simulink model "Ladder_Model"  (R2021b)
settings: Solver=VariableStepAuto  StartTime=0.0  StopTime=0.00005  RelTol=1e-3
model workspace (MAT data in the model file):
  f = [1 10010011.009 20020021.018 30030031.027 40040041.036 50050051.045 60060061.0541 70070071.0631 80080081.0721 90090091.0811 100100101.09 110110111.099 ... (1000 elements, 1x1000)]
  f1 = 120
  fff : Simulink.Parameter (value not decoded)
undefined symbols (not defined in the file or in its folder): c0, ct0, ct1, ct2, ct3, ct4, cu, cv, frequence
libraries: spsSeriesRLCBranchLib x190, spsGroundLib x49, spsControlledVoltageSourceLib x6, spsImpedanceMeasurementLib x6, spspowerguiLib x1
(part 2 of 2)

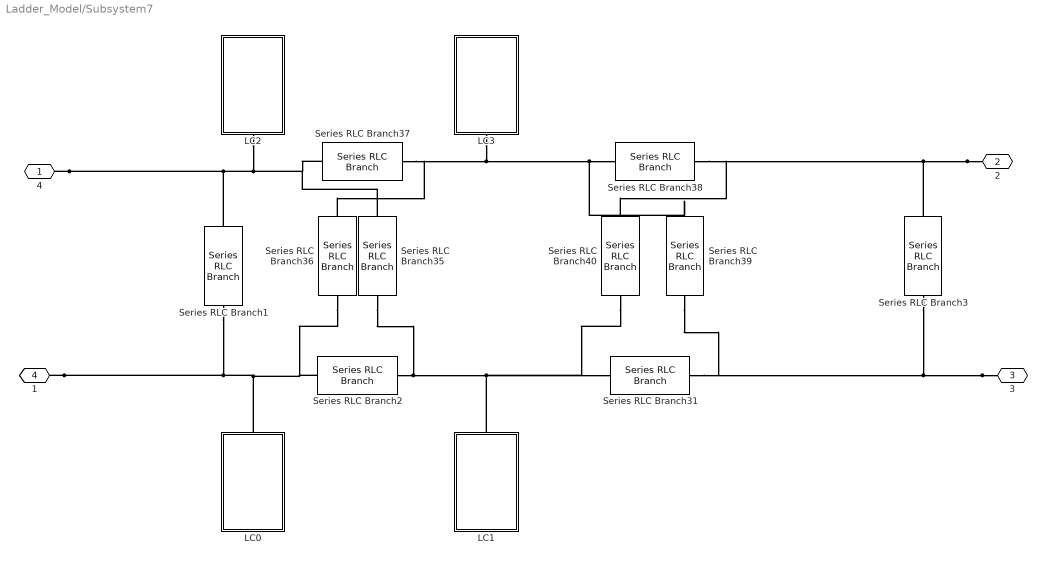
== system Ladder_Model/Subsystem7 ==
  LC0 : Subsystem
  LC1 : Subsystem
  LC2 : Subsystem
  LC3 : Subsystem
  Series RLC Branch1 : spsSeriesRLCBranchLib/Series RLC Branch  LConnTagsString=__new0  RConnTagsString=__new0  BranchType=C  Resistance=1  Inductance=1e-6  SetiL0=off  InitialCurrent=0  Capacitance=ct0  Setx0=off  InitialVoltage=0  Measurements=None
  Series RLC Branch2 : spsSeriesRLCBranchLib/Series RLC Branch  LConnTagsString=__new0  RConnTagsString=__new0  BranchType=C  Resistance=1  Inductance=1e-6  SetiL0=off  InitialCurrent=0  Capacitance=cu  Setx0=off  InitialVoltage=0  Measurements=None
  Series RLC Branch3 : spsSeriesRLCBranchLib/Series RLC Branch  LConnTagsString=__new0  RConnTagsString=__new0  BranchType=C  Resistance=1  Inductance=1e-6  SetiL0=off  InitialCurrent=0  Capacitance=ct0  Setx0=off  InitialVoltage=0  Measurements=None
  Series RLC Branch31 : spsSeriesRLCBranchLib/Series RLC Branch  LConnTagsString=__new0  RConnTagsString=__new0  BranchType=C  Resistance=1  Inductance=1e-6  SetiL0=off  InitialCurrent=0  Capacitance=cv  Setx0=off  InitialVoltage=0  Measurements=None
  Series RLC Branch35 : spsSeriesRLCBranchLib/Series RLC Branch  LConnTagsString=__new0  RConnTagsString=__new0  BranchType=C  Resistance=1  Inductance=1e-6  SetiL0=off  InitialCurrent=0  Capacitance=ct2  Setx0=off  InitialVoltage=0  Measurements=None
  Series RLC Branch36 : spsSeriesRLCBranchLib/Series RLC Branch  LConnTagsString=__new0  RConnTagsString=__new0  BranchType=C  Resistance=1  Inductance=1e-6  SetiL0=off  InitialCurrent=0  Capacitance=ct1  Setx0=off  InitialVoltage=0  Measurements=None
  Series RLC Branch37 : spsSeriesRLCBranchLib/Series RLC Branch  LConnTagsString=__new0  RConnTagsString=__new0  BranchType=C  Resistance=1  Inductance=1e-6  SetiL0=off  InitialCurrent=0  Capacitance=cu  Setx0=off  InitialVoltage=0  Measurements=None
  Series RLC Branch38 : spsSeriesRLCBranchLib/Series RLC Branch  LConnTagsString=__new0  RConnTagsString=__new0  BranchType=C  Resistance=1  Inductance=1e-6  SetiL0=off  InitialCurrent=0  Capacitance=cv  Setx0=off  InitialVoltage=0  Measurements=None
  Series RLC Branch39 : spsSeriesRLCBranchLib/Series RLC Branch  LConnTagsString=__new0  RConnTagsString=__new0  BranchType=C  Resistance=1  Inductance=1e-6  SetiL0=off  InitialCurrent=0  Capacitance=ct4  Setx0=off  InitialVoltage=0  Measurements=None
  Series RLC Branch40 : spsSeriesRLCBranchLib/Series RLC Branch  LConnTagsString=__new0  RConnTagsString=__new0  BranchType=C  Resistance=1  Inductance=1e-6  SetiL0=off  InitialCurrent=0  Capacitance=ct3  Setx0=off  InitialVoltage=0  Measurements=None
  4 : PMIOPort  Side=Left
  2 : PMIOPort  Port=2  Side=Right
  3 : PMIOPort  Port=3  Side=Right
  1 : PMIOPort  Port=4  Side=Left
  connections:
  3/RConn1 -- Series RLC Branch39/RConn1 -- Series RLC Branch31/RConn1 -- Series RLC Branch3/LConn1
  Series RLC Branch39/LConn1 -- Series RLC Branch38/LConn1 -- Series RLC Branch37/RConn1 -- Series RLC Branch36/RConn1 -- LC3/LConn1
  4/RConn1 -- Series RLC Branch37/LConn1 -- Series RLC Branch35/LConn1 -- LC2/LConn1 -- Series RLC Branch1/RConn1
  Series RLC Branch35/RConn1 -- Series RLC Branch2/RConn1 -- LC1/LConn1 -- Series RLC Branch40/LConn1 -- Series RLC Branch31/LConn1
  2/RConn1 -- Series RLC Branch40/RConn1 -- Series RLC Branch38/RConn1 -- Series RLC Branch3/RConn1
  1/RConn1 -- Series RLC Branch36/LConn1 -- Series RLC Branch2/LConn1 -- LC0/LConn1 -- Series RLC Branch1/LConn1

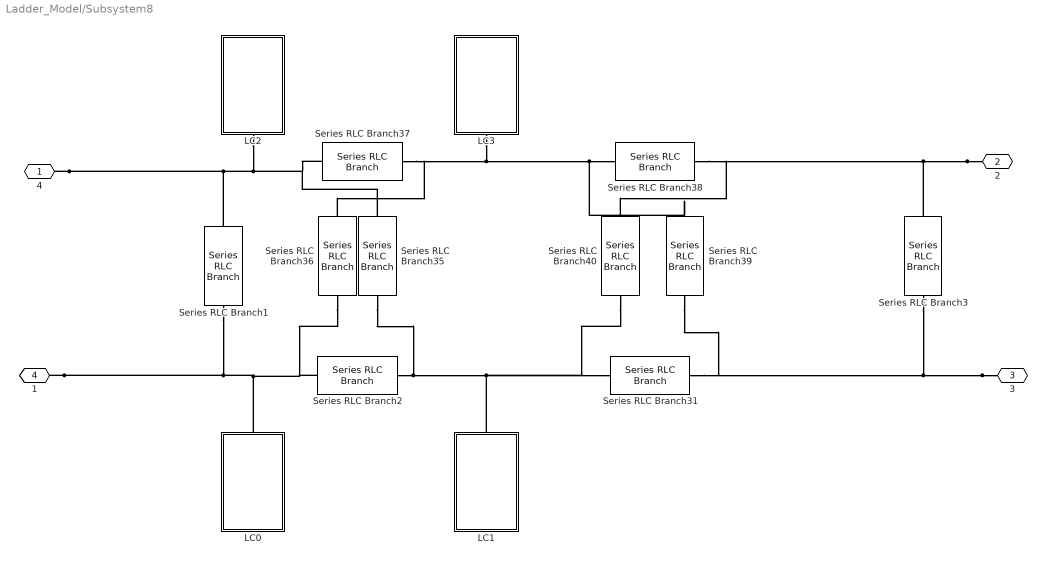
== system Ladder_Model/Subsystem8 ==
  LC0 : Subsystem
  LC1 : Subsystem
  LC2 : Subsystem
  LC3 : Subsystem
  Series RLC Branch1 : spsSeriesRLCBranchLib/Series RLC Branch  LConnTagsString=__new0  RConnTagsString=__new0  BranchType=C  Resistance=1  Inductance=1e-6  SetiL0=off  InitialCurrent=0  Capacitance=ct0  Setx0=off  InitialVoltage=0  Measurements=None
  Series RLC Branch2 : spsSeriesRLCBranchLib/Series RLC Branch  LConnTagsString=__new0  RConnTagsString=__new0  BranchType=C  Resistance=1  Inductance=1e-6  SetiL0=off  InitialCurrent=0  Capacitance=cu  Setx0=off  InitialVoltage=0  Measurements=None
  Series RLC Branch3 : spsSeriesRLCBranchLib/Series RLC Branch  LConnTagsString=__new0  RConnTagsString=__new0  BranchType=C  Resistance=1  Inductance=1e-6  SetiL0=off  InitialCurrent=0  Capacitance=ct0  Setx0=off  InitialVoltage=0  Measurements=None
  Series RLC Branch31 : spsSeriesRLCBranchLib/Series RLC Branch  LConnTagsString=__new0  RConnTagsString=__new0  BranchType=C  Resistance=1  Inductance=1e-6  SetiL0=off  InitialCurrent=0  Capacitance=cv  Setx0=off  InitialVoltage=0  Measurements=None
  Series RLC Branch35 : spsSeriesRLCBranchLib/Series RLC Branch  LConnTagsString=__new0  RConnTagsString=__new0  BranchType=C  Resistance=1  Inductance=1e-6  SetiL0=off  InitialCurrent=0  Capacitance=ct2  Setx0=off  InitialVoltage=0  Measurements=None
  Series RLC Branch36 : spsSeriesRLCBranchLib/Series RLC Branch  LConnTagsString=__new0  RConnTagsString=__new0  BranchType=C  Resistance=1  Inductance=1e-6  SetiL0=off  InitialCurrent=0  Capacitance=ct1  Setx0=off  InitialVoltage=0  Measurements=None
  Series RLC Branch37 : spsSeriesRLCBranchLib/Series RLC Branch  LConnTagsString=__new0  RConnTagsString=__new0  BranchType=C  Resistance=1  Inductance=1e-6  SetiL0=off  InitialCurrent=0  Capacitance=cu  Setx0=off  InitialVoltage=0  Measurements=None
  Series RLC Branch38 : spsSeriesRLCBranchLib/Series RLC Branch  LConnTagsString=__new0  RConnTagsString=__new0  BranchType=C  Resistance=1  Inductance=1e-6  SetiL0=off  InitialCurrent=0  Capacitance=cv  Setx0=off  InitialVoltage=0  Measurements=None
  Series RLC Branch39 : spsSeriesRLCBranchLib/Series RLC Branch  LConnTagsString=__new0  RConnTagsString=__new0  BranchType=C  Resistance=1  Inductance=1e-6  SetiL0=off  InitialCurrent=0  Capacitance=ct4  Setx0=off  InitialVoltage=0  Measurements=None
  Series RLC Branch40 : spsSeriesRLCBranchLib/Series RLC Branch  LConnTagsString=__new0  RConnTagsString=__new0  BranchType=C  Resistance=1  Inductance=1e-6  SetiL0=off  InitialCurrent=0  Capacitance=ct3  Setx0=off  InitialVoltage=0  Measurements=None
  4 : PMIOPort  Side=Left
  2 : PMIOPort  Port=2  Side=Right
  3 : PMIOPort  Port=3  Side=Right
  1 : PMIOPort  Port=4  Side=Left
  connections:
  3/RConn1 -- Series RLC Branch39/RConn1 -- Series RLC Branch31/RConn1 -- Series RLC Branch3/LConn1
  Series RLC Branch39/LConn1 -- Series RLC Branch38/LConn1 -- Series RLC Branch37/RConn1 -- Series RLC Branch36/RConn1 -- LC3/LConn1
  4/RConn1 -- Series RLC Branch37/LConn1 -- Series RLC Branch35/LConn1 -- LC2/LConn1 -- Series RLC Branch1/RConn1
  Series RLC Branch35/RConn1 -- Series RLC Branch2/RConn1 -- LC1/LConn1 -- Series RLC Branch40/LConn1 -- Series RLC Branch31/LConn1
  2/RConn1 -- Series RLC Branch40/RConn1 -- Series RLC Branch38/RConn1 -- Series RLC Branch3/RConn1
  1/RConn1 -- Series RLC Branch36/LConn1 -- Series RLC Branch2/LConn1 -- LC0/LConn1 -- Series RLC Branch1/LConn1

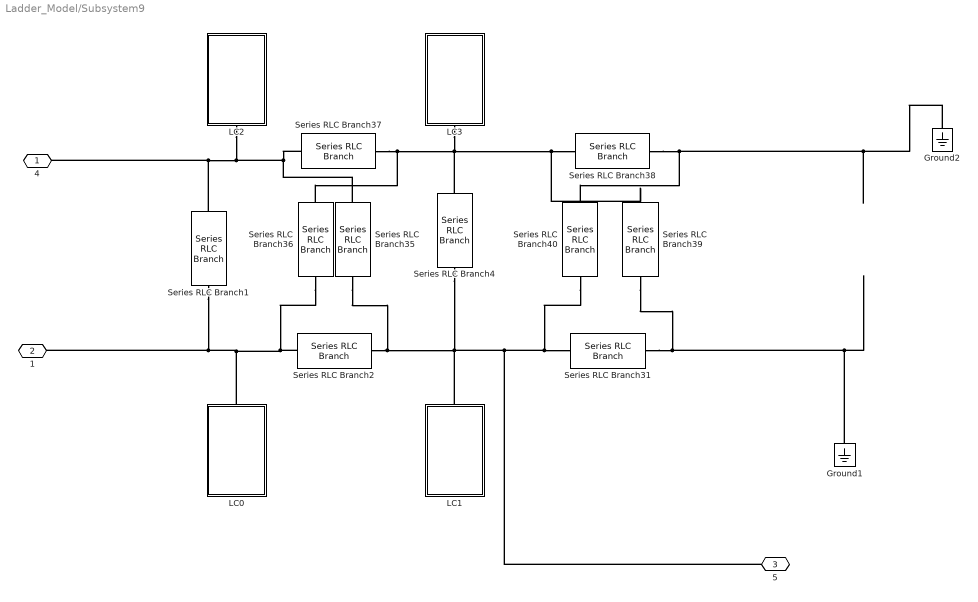
== system Ladder_Model/Subsystem9 ==
  Ground1 : spsGroundLib/Ground  LConnTagsString=a
  Ground2 : spsGroundLib/Ground  LConnTagsString=a
  LC0 : Subsystem
  LC1 : Subsystem
  LC2 : Subsystem
  LC3 : Subsystem
  Series RLC Branch1 : spsSeriesRLCBranchLib/Series RLC Branch  LConnTagsString=__new0  RConnTagsString=__new0  BranchType=C  Resistance=1  Inductance=1e-6  SetiL0=off  InitialCurrent=0  Capacitance=ct0  Setx0=off  InitialVoltage=0  Measurements=None
  Series RLC Branch2 : spsSeriesRLCBranchLib/Series RLC Branch  LConnTagsString=__new0  RConnTagsString=__new0  BranchType=C  Resistance=1  Inductance=1e-6  SetiL0=off  InitialCurrent=0  Capacitance=cu  Setx0=off  InitialVoltage=0  Measurements=None
  Series RLC Branch31 : spsSeriesRLCBranchLib/Series RLC Branch  LConnTagsString=__new0  RConnTagsString=__new0  BranchType=C  Resistance=1  Inductance=1e-6  SetiL0=off  InitialCurrent=0  Capacitance=cv  Setx0=off  InitialVoltage=0  Measurements=None
  Series RLC Branch35 : spsSeriesRLCBranchLib/Series RLC Branch  LConnTagsString=__new0  RConnTagsString=__new0  BranchType=C  Resistance=1  Inductance=1e-6  SetiL0=off  InitialCurrent=0  Capacitance=ct2  Setx0=off  InitialVoltage=0  Measurements=None
  Series RLC Branch36 : spsSeriesRLCBranchLib/Series RLC Branch  LConnTagsString=__new0  RConnTagsString=__new0  BranchType=C  Resistance=1  Inductance=1e-6  SetiL0=off  InitialCurrent=0  Capacitance=ct1  Setx0=off  InitialVoltage=0  Measurements=None
  Series RLC Branch37 : spsSeriesRLCBranchLib/Series RLC Branch  LConnTagsString=__new0  RConnTagsString=__new0  BranchType=C  Resistance=1  Inductance=1e-6  SetiL0=off  InitialCurrent=0  Capacitance=cu  Setx0=off  InitialVoltage=0  Measurements=None
  Series RLC Branch38 : spsSeriesRLCBranchLib/Series RLC Branch  LConnTagsString=__new0  RConnTagsString=__new0  BranchType=C  Resistance=1  Inductance=1e-6  SetiL0=off  InitialCurrent=0  Capacitance=cv  Setx0=off  InitialVoltage=0  Measurements=None
  Series RLC Branch39 : spsSeriesRLCBranchLib/Series RLC Branch  LConnTagsString=__new0  RConnTagsString=__new0  BranchType=C  Resistance=1  Inductance=1e-6  SetiL0=off  InitialCurrent=0  Capacitance=ct4  Setx0=off  InitialVoltage=0  Measurements=None
  Series RLC Branch4 : spsSeriesRLCBranchLib/Series RLC Branch  LConnTagsString=__new0  RConnTagsString=__new0  BranchType=C  Resistance=1  Inductance=1e-6  SetiL0=off  InitialCurrent=0  Capacitance=ct0  Setx0=off  InitialVoltage=0  Measurements=None
  Series RLC Branch40 : spsSeriesRLCBranchLib/Series RLC Branch  LConnTagsString=__new0  RConnTagsString=__new0  BranchType=C  Resistance=1  Inductance=1e-6  SetiL0=off  InitialCurrent=0  Capacitance=ct3  Setx0=off  InitialVoltage=0  Measurements=None
  4 : PMIOPort  Side=Left
  1 : PMIOPort  Port=2  Side=Left
  5 : PMIOPort  Port=3  Side=Right
  connections:
  Series RLC Branch39/RConn1 -- Ground1/LConn1 -- Series RLC Branch31/RConn1
  Series RLC Branch39/LConn1 -- Series RLC Branch4/RConn1 -- Series RLC Branch37/RConn1 -- Series RLC Branch36/RConn1 -- LC3/LConn1 -- Series RLC Branch38/LConn1
  4/RConn1 -- Series RLC Branch37/LConn1 -- Series RLC Branch35/LConn1 -- LC2/LConn1 -- Series RLC Branch1/RConn1
  Series RLC Branch35/RConn1 -- Series RLC Branch2/RConn1 -- Series RLC Branch4/LConn1 -- 5/RConn1 -- Series RLC Branch40/LConn1 -- Series RLC Branch31/LConn1 -- LC1/LConn1
  Series RLC Branch40/RConn1 -- Ground2/LConn1 -- Series RLC Branch38/RConn1
  1/RConn1 -- Series RLC Branch36/LConn1 -- Series RLC Branch2/LConn1 -- LC0/LConn1 -- Series RLC Branch1/LConn1

== system Ladder_Model/Subsystem/LC0 ==
  Ground : spsGroundLib/Ground  LConnTagsString=a
  Series RLC Branch2 : spsSeriesRLCBranchLib/Series RLC Branch  LConnTagsString=__new0  RConnTagsString=__new0  BranchType=L  Resistance=1  Inductance=1e-6  SetiL0=off  InitialCurrent=0  Capacitance=1e-6  Setx0=off  InitialVoltage=0  Measurements=None
  Series RLC Branch31 : spsSeriesRLCBranchLib/Series RLC Branch  LConnTagsString=__new0  RConnTagsString=__new0  BranchType=C  Resistance=1  Inductance=1e-6  SetiL0=off  InitialCurrent=0  Capacitance=c0  Setx0=off  InitialVoltage=0  Measurements=None
  Conn1 : PMIOPort  Side=Left
  connections:
  Series RLC Branch2/LConn1 -- Conn1/RConn1 -- Series RLC Branch31/LConn1
  Series RLC Branch2/RConn1 -- Ground/LConn1 -- Series RLC Branch31/RConn1

== system Ladder_Model/Subsystem/LC1 ==
  Ground : spsGroundLib/Ground  LConnTagsString=a
  Series RLC Branch2 : spsSeriesRLCBranchLib/Series RLC Branch  LConnTagsString=__new0  RConnTagsString=__new0  BranchType=L  Resistance=1  Inductance=1e-6  SetiL0=off  InitialCurrent=0  Capacitance=1e-6  Setx0=off  InitialVoltage=0  Measurements=None
  Series RLC Branch31 : spsSeriesRLCBranchLib/Series RLC Branch  LConnTagsString=__new0  RConnTagsString=__new0  BranchType=C  Resistance=1  Inductance=1e-6  SetiL0=off  InitialCurrent=0  Capacitance=c0  Setx0=off  InitialVoltage=0  Measurements=None
  Conn1 : PMIOPort  Side=Left
  connections:
  Series RLC Branch31/LConn1 -- Series RLC Branch2/LConn1 -- Conn1/RConn1
  Series RLC Branch31/RConn1 -- Series RLC Branch2/RConn1 -- Ground/LConn1

== system Ladder_Model/Subsystem/LC2 ==
  Ground : spsGroundLib/Ground  LConnTagsString=a
  Series RLC Branch2 : spsSeriesRLCBranchLib/Series RLC Branch  LConnTagsString=__new0  RConnTagsString=__new0  BranchType=L  Resistance=1  Inductance=1e-6  SetiL0=off  InitialCurrent=0  Capacitance=1e-6  Setx0=off  InitialVoltage=0  Measurements=None
  Series RLC Branch31 : spsSeriesRLCBranchLib/Series RLC Branch  LConnTagsString=__new0  RConnTagsString=__new0  BranchType=C  Resistance=1  Inductance=1e-6  SetiL0=off  InitialCurrent=0  Capacitance=c0  Setx0=off  InitialVoltage=0  Measurements=None
  Conn1 : PMIOPort  Side=Left
  connections:
  Series RLC Branch31/LConn1 -- Series RLC Branch2/LConn1 -- Conn1/RConn1
  Series RLC Branch31/RConn1 -- Series RLC Branch2/RConn1 -- Ground/LConn1

== system Ladder_Model/Subsystem/LC3 ==
  Ground : spsGroundLib/Ground  LConnTagsString=a
  Series RLC Branch2 : spsSeriesRLCBranchLib/Series RLC Branch  LConnTagsString=__new0  RConnTagsString=__new0  BranchType=L  Resistance=1  Inductance=1e-6  SetiL0=off  InitialCurrent=0  Capacitance=1e-6  Setx0=off  InitialVoltage=0  Measurements=None
  Series RLC Branch31 : spsSeriesRLCBranchLib/Series RLC Branch  LConnTagsString=__new0  RConnTagsString=__new0  BranchType=C  Resistance=1  Inductance=1e-6  SetiL0=off  InitialCurrent=0  Capacitance=c0  Setx0=off  InitialVoltage=0  Measurements=None
  Conn1 : PMIOPort  Side=Left
  connections:
  Series RLC Branch31/LConn1 -- Series RLC Branch2/LConn1 -- Conn1/RConn1
  Series RLC Branch31/RConn1 -- Series RLC Branch2/RConn1 -- Ground/LConn1

== system Ladder_Model/Subsystem1/LC0 ==
  Ground : spsGroundLib/Ground  LConnTagsString=a
  Series RLC Branch2 : spsSeriesRLCBranchLib/Series RLC Branch  LConnTagsString=__new0  RConnTagsString=__new0  BranchType=L  Resistance=1  Inductance=1e-6  SetiL0=off  InitialCurrent=0  Capacitance=1e-6  Setx0=off  InitialVoltage=0  Measurements=None
  Series RLC Branch31 : spsSeriesRLCBranchLib/Series RLC Branch  LConnTagsString=__new0  RConnTagsString=__new0  BranchType=C  Resistance=1  Inductance=1e-6  SetiL0=off  InitialCurrent=0  Capacitance=c0  Setx0=off  InitialVoltage=0  Measurements=None
  Conn1 : PMIOPort  Side=Left
  connections:
  Series RLC Branch31/LConn1 -- Series RLC Branch2/LConn1 -- Conn1/RConn1
  Series RLC Branch31/RConn1 -- Series RLC Branch2/RConn1 -- Ground/LConn1

== system Ladder_Model/Subsystem1/LC1 ==
  Ground : spsGroundLib/Ground  LConnTagsString=a
  Series RLC Branch2 : spsSeriesRLCBranchLib/Series RLC Branch  LConnTagsString=__new0  RConnTagsString=__new0  BranchType=L  Resistance=1  Inductance=1e-6  SetiL0=off  InitialCurrent=0  Capacitance=1e-6  Setx0=off  InitialVoltage=0  Measurements=None
  Series RLC Branch31 : spsSeriesRLCBranchLib/Series RLC Branch  LConnTagsString=__new0  RConnTagsString=__new0  BranchType=C  Resistance=1  Inductance=1e-6  SetiL0=off  InitialCurrent=0  Capacitance=c0  Setx0=off  InitialVoltage=0  Measurements=None
  Conn1 : PMIOPort  Side=Left
  connections:
  Series RLC Branch31/LConn1 -- Series RLC Branch2/LConn1 -- Conn1/RConn1
  Series RLC Branch31/RConn1 -- Series RLC Branch2/RConn1 -- Ground/LConn1

== system Ladder_Model/Subsystem1/LC2 ==
  Ground : spsGroundLib/Ground  LConnTagsString=a
  Series RLC Branch2 : spsSeriesRLCBranchLib/Series RLC Branch  LConnTagsString=__new0  RConnTagsString=__new0  BranchType=L  Resistance=1  Inductance=1e-6  SetiL0=off  InitialCurrent=0  Capacitance=1e-6  Setx0=off  InitialVoltage=0  Measurements=None
  Series RLC Branch31 : spsSeriesRLCBranchLib/Series RLC Branch  LConnTagsString=__new0  RConnTagsString=__new0  BranchType=C  Resistance=1  Inductance=1e-6  SetiL0=off  InitialCurrent=0  Capacitance=c0  Setx0=off  InitialVoltage=0  Measurements=None
  Conn1 : PMIOPort  Side=Left
  connections:
  Series RLC Branch31/LConn1 -- Series RLC Branch2/LConn1 -- Conn1/RConn1
  Series RLC Branch31/RConn1 -- Series RLC Branch2/RConn1 -- Ground/LConn1

== system Ladder_Model/Subsystem1/LC3 ==
  Ground : spsGroundLib/Ground  LConnTagsString=a
  Series RLC Branch2 : spsSeriesRLCBranchLib/Series RLC Branch  LConnTagsString=__new0  RConnTagsString=__new0  BranchType=L  Resistance=1  Inductance=1e-6  SetiL0=off  InitialCurrent=0  Capacitance=1e-6  Setx0=off  InitialVoltage=0  Measurements=None
  Series RLC Branch31 : spsSeriesRLCBranchLib/Series RLC Branch  LConnTagsString=__new0  RConnTagsString=__new0  BranchType=C  Resistance=1  Inductance=1e-6  SetiL0=off  InitialCurrent=0  Capacitance=c0  Setx0=off  InitialVoltage=0  Measurements=None
  Conn1 : PMIOPort  Side=Left
  connections:
  Series RLC Branch31/LConn1 -- Series RLC Branch2/LConn1 -- Conn1/RConn1
  Series RLC Branch31/RConn1 -- Series RLC Branch2/RConn1 -- Ground/LConn1

== system Ladder_Model/Subsystem2/LC0 ==
  Ground : spsGroundLib/Ground  LConnTagsString=a
  Series RLC Branch2 : spsSeriesRLCBranchLib/Series RLC Branch  LConnTagsString=__new0  RConnTagsString=__new0  BranchType=L  Resistance=1  Inductance=1e-6  SetiL0=off  InitialCurrent=0  Capacitance=1e-6  Setx0=off  InitialVoltage=0  Measurements=None
  Series RLC Branch31 : spsSeriesRLCBranchLib/Series RLC Branch  LConnTagsString=__new0  RConnTagsString=__new0  BranchType=C  Resistance=1  Inductance=1e-6  SetiL0=off  InitialCurrent=0  Capacitance=c0  Setx0=off  InitialVoltage=0  Measurements=None
  Conn1 : PMIOPort  Side=Left
  connections:
  Series RLC Branch31/LConn1 -- Series RLC Branch2/LConn1 -- Conn1/RConn1
  Series RLC Branch31/RConn1 -- Series RLC Branch2/RConn1 -- Ground/LConn1

== system Ladder_Model/Subsystem2/LC1 ==
  Ground : spsGroundLib/Ground  LConnTagsString=a
  Series RLC Branch2 : spsSeriesRLCBranchLib/Series RLC Branch  LConnTagsString=__new0  RConnTagsString=__new0  BranchType=L  Resistance=1  Inductance=1e-6  SetiL0=off  InitialCurrent=0  Capacitance=1e-6  Setx0=off  InitialVoltage=0  Measurements=None
  Series RLC Branch31 : spsSeriesRLCBranchLib/Series RLC Branch  LConnTagsString=__new0  RConnTagsString=__new0  BranchType=C  Resistance=1  Inductance=1e-6  SetiL0=off  InitialCurrent=0  Capacitance=c0  Setx0=off  InitialVoltage=0  Measurements=None
  Conn1 : PMIOPort  Side=Left
  connections:
  Series RLC Branch31/LConn1 -- Series RLC Branch2/LConn1 -- Conn1/RConn1
  Series RLC Branch31/RConn1 -- Series RLC Branch2/RConn1 -- Ground/LConn1

== system Ladder_Model/Subsystem2/LC2 ==
  Ground : spsGroundLib/Ground  LConnTagsString=a
  Series RLC Branch2 : spsSeriesRLCBranchLib/Series RLC Branch  LConnTagsString=__new0  RConnTagsString=__new0  BranchType=L  Resistance=1  Inductance=1e-6  SetiL0=off  InitialCurrent=0  Capacitance=1e-6  Setx0=off  InitialVoltage=0  Measurements=None
  Series RLC Branch31 : spsSeriesRLCBranchLib/Series RLC Branch  LConnTagsString=__new0  RConnTagsString=__new0  BranchType=C  Resistance=1  Inductance=1e-6  SetiL0=off  InitialCurrent=0  Capacitance=c0  Setx0=off  InitialVoltage=0  Measurements=None
  Conn1 : PMIOPort  Side=Left
  connections:
  Series RLC Branch31/LConn1 -- Series RLC Branch2/LConn1 -- Conn1/RConn1
  Series RLC Branch31/RConn1 -- Series RLC Branch2/RConn1 -- Ground/LConn1

== system Ladder_Model/Subsystem2/LC3 ==
  Ground : spsGroundLib/Ground  LConnTagsString=a
  Series RLC Branch2 : spsSeriesRLCBranchLib/Series RLC Branch  LConnTagsString=__new0  RConnTagsString=__new0  BranchType=L  Resistance=1  Inductance=1e-6  SetiL0=off  InitialCurrent=0  Capacitance=1e-6  Setx0=off  InitialVoltage=0  Measurements=None
  Series RLC Branch31 : spsSeriesRLCBranchLib/Series RLC Branch  LConnTagsString=__new0  RConnTagsString=__new0  BranchType=C  Resistance=1  Inductance=1e-6  SetiL0=off  InitialCurrent=0  Capacitance=c0  Setx0=off  InitialVoltage=0  Measurements=None
  Conn1 : PMIOPort  Side=Left
  connections:
  Series RLC Branch31/LConn1 -- Series RLC Branch2/LConn1 -- Conn1/RConn1
  Series RLC Branch31/RConn1 -- Series RLC Branch2/RConn1 -- Ground/LConn1

== system Ladder_Model/Subsystem3/LC0 ==
  Ground : spsGroundLib/Ground  LConnTagsString=a
  Series RLC Branch2 : spsSeriesRLCBranchLib/Series RLC Branch  LConnTagsString=__new0  RConnTagsString=__new0  BranchType=L  Resistance=1  Inductance=1e-6  SetiL0=off  InitialCurrent=0  Capacitance=1e-6  Setx0=off  InitialVoltage=0  Measurements=None
  Series RLC Branch31 : spsSeriesRLCBranchLib/Series RLC Branch  LConnTagsString=__new0  RConnTagsString=__new0  BranchType=C  Resistance=1  Inductance=1e-6  SetiL0=off  InitialCurrent=0  Capacitance=c0  Setx0=off  InitialVoltage=0  Measurements=None
  Conn1 : PMIOPort  Side=Left
  connections:
  Series RLC Branch31/LConn1 -- Series RLC Branch2/LConn1 -- Conn1/RConn1
  Series RLC Branch31/RConn1 -- Series RLC Branch2/RConn1 -- Ground/LConn1

== system Ladder_Model/Subsystem3/LC1 ==
  Ground : spsGroundLib/Ground  LConnTagsString=a
  Series RLC Branch2 : spsSeriesRLCBranchLib/Series RLC Branch  LConnTagsString=__new0  RConnTagsString=__new0  BranchType=L  Resistance=1  Inductance=1e-6  SetiL0=off  InitialCurrent=0  Capacitance=1e-6  Setx0=off  InitialVoltage=0  Measurements=None
  Series RLC Branch31 : spsSeriesRLCBranchLib/Series RLC Branch  LConnTagsString=__new0  RConnTagsString=__new0  BranchType=C  Resistance=1  Inductance=1e-6  SetiL0=off  InitialCurrent=0  Capacitance=c0  Setx0=off  InitialVoltage=0  Measurements=None
  Conn1 : PMIOPort  Side=Left
  connections:
  Series RLC Branch31/LConn1 -- Series RLC Branch2/LConn1 -- Conn1/RConn1
  Series RLC Branch31/RConn1 -- Series RLC Branch2/RConn1 -- Ground/LConn1

== system Ladder_Model/Subsystem3/LC2 ==
  Ground : spsGroundLib/Ground  LConnTagsString=a
  Series RLC Branch2 : spsSeriesRLCBranchLib/Series RLC Branch  LConnTagsString=__new0  RConnTagsString=__new0  BranchType=L  Resistance=1  Inductance=1e-6  SetiL0=off  InitialCurrent=0  Capacitance=1e-6  Setx0=off  InitialVoltage=0  Measurements=None
  Series RLC Branch31 : spsSeriesRLCBranchLib/Series RLC Branch  LConnTagsString=__new0  RConnTagsString=__new0  BranchType=C  Resistance=1  Inductance=1e-6  SetiL0=off  InitialCurrent=0  Capacitance=c0  Setx0=off  InitialVoltage=0  Measurements=None
  Conn1 : PMIOPort  Side=Left
  connections:
  Series RLC Branch31/LConn1 -- Series RLC Branch2/LConn1 -- Conn1/RConn1
  Series RLC Branch31/RConn1 -- Series RLC Branch2/RConn1 -- Ground/LConn1

== system Ladder_Model/Subsystem3/LC3 ==
  Ground : spsGroundLib/Ground  LConnTagsString=a
  Series RLC Branch2 : spsSeriesRLCBranchLib/Series RLC Branch  LConnTagsString=__new0  RConnTagsString=__new0  BranchType=L  Resistance=1  Inductance=1e-6  SetiL0=off  InitialCurrent=0  Capacitance=1e-6  Setx0=off  InitialVoltage=0  Measurements=None
  Series RLC Branch31 : spsSeriesRLCBranchLib/Series RLC Branch  LConnTagsString=__new0  RConnTagsString=__new0  BranchType=C  Resistance=1  Inductance=1e-6  SetiL0=off  InitialCurrent=0  Capacitance=c0  Setx0=off  InitialVoltage=0  Measurements=None
  Conn1 : PMIOPort  Side=Left
  connections:
  Series RLC Branch31/LConn1 -- Series RLC Branch2/LConn1 -- Conn1/RConn1
  Series RLC Branch31/RConn1 -- Series RLC Branch2/RConn1 -- Ground/LConn1

== system Ladder_Model/Subsystem4/LC0 ==
  Ground : spsGroundLib/Ground  LConnTagsString=a
  Series RLC Branch2 : spsSeriesRLCBranchLib/Series RLC Branch  LConnTagsString=__new0  RConnTagsString=__new0  BranchType=L  Resistance=1  Inductance=1e-6  SetiL0=off  InitialCurrent=0  Capacitance=1e-6  Setx0=off  InitialVoltage=0  Measurements=None
  Series RLC Branch31 : spsSeriesRLCBranchLib/Series RLC Branch  LConnTagsString=__new0  RConnTagsString=__new0  BranchType=C  Resistance=1  Inductance=1e-6  SetiL0=off  InitialCurrent=0  Capacitance=c0  Setx0=off  InitialVoltage=0  Measurements=None
  Conn1 : PMIOPort  Side=Left
  connections:
  Series RLC Branch31/LConn1 -- Series RLC Branch2/LConn1 -- Conn1/RConn1
  Series RLC Branch31/RConn1 -- Series RLC Branch2/RConn1 -- Ground/LConn1

== system Ladder_Model/Subsystem4/LC1 ==
  Ground : spsGroundLib/Ground  LConnTagsString=a
  Series RLC Branch2 : spsSeriesRLCBranchLib/Series RLC Branch  LConnTagsString=__new0  RConnTagsString=__new0  BranchType=L  Resistance=1  Inductance=1e-6  SetiL0=off  InitialCurrent=0  Capacitance=1e-6  Setx0=off  InitialVoltage=0  Measurements=None
  Series RLC Branch31 : spsSeriesRLCBranchLib/Series RLC Branch  LConnTagsString=__new0  RConnTagsString=__new0  BranchType=C  Resistance=1  Inductance=1e-6  SetiL0=off  InitialCurrent=0  Capacitance=c0  Setx0=off  InitialVoltage=0  Measurements=None
  Conn1 : PMIOPort  Side=Left
  connections:
  Series RLC Branch31/LConn1 -- Series RLC Branch2/LConn1 -- Conn1/RConn1
  Series RLC Branch31/RConn1 -- Series RLC Branch2/RConn1 -- Ground/LConn1

== system Ladder_Model/Subsystem4/LC2 ==
  Ground : spsGroundLib/Ground  LConnTagsString=a
  Series RLC Branch2 : spsSeriesRLCBranchLib/Series RLC Branch  LConnTagsString=__new0  RConnTagsString=__new0  BranchType=L  Resistance=1  Inductance=1e-6  SetiL0=off  InitialCurrent=0  Capacitance=1e-6  Setx0=off  InitialVoltage=0  Measurements=None
  Series RLC Branch31 : spsSeriesRLCBranchLib/Series RLC Branch  LConnTagsString=__new0  RConnTagsString=__new0  BranchType=C  Resistance=1  Inductance=1e-6  SetiL0=off  InitialCurrent=0  Capacitance=c0  Setx0=off  InitialVoltage=0  Measurements=None
  Conn1 : PMIOPort  Side=Left
  connections:
  Series RLC Branch31/LConn1 -- Series RLC Branch2/LConn1 -- Conn1/RConn1
  Series RLC Branch31/RConn1 -- Series RLC Branch2/RConn1 -- Ground/LConn1

== system Ladder_Model/Subsystem4/LC3 ==
  Ground : spsGroundLib/Ground  LConnTagsString=a
  Series RLC Branch2 : spsSeriesRLCBranchLib/Series RLC Branch  LConnTagsString=__new0  RConnTagsString=__new0  BranchType=L  Resistance=1  Inductance=1e-6  SetiL0=off  InitialCurrent=0  Capacitance=1e-6  Setx0=off  InitialVoltage=0  Measurements=None
  Series RLC Branch31 : spsSeriesRLCBranchLib/Series RLC Branch  LConnTagsString=__new0  RConnTagsString=__new0  BranchType=C  Resistance=1  Inductance=1e-6  SetiL0=off  InitialCurrent=0  Capacitance=c0  Setx0=off  InitialVoltage=0  Measurements=None
  Conn1 : PMIOPort  Side=Left
  connections:
  Series RLC Branch31/LConn1 -- Series RLC Branch2/LConn1 -- Conn1/RConn1
  Series RLC Branch31/RConn1 -- Series RLC Branch2/RConn1 -- Ground/LConn1

== system Ladder_Model/Subsystem5/LC0 ==
  Ground : spsGroundLib/Ground  LConnTagsString=a
  Series RLC Branch2 : spsSeriesRLCBranchLib/Series RLC Branch  LConnTagsString=__new0  RConnTagsString=__new0  BranchType=L  Resistance=1  Inductance=1e-6  SetiL0=off  InitialCurrent=0  Capacitance=1e-6  Setx0=off  InitialVoltage=0  Measurements=None
  Series RLC Branch31 : spsSeriesRLCBranchLib/Series RLC Branch  LConnTagsString=__new0  RConnTagsString=__new0  BranchType=C  Resistance=1  Inductance=1e-6  SetiL0=off  InitialCurrent=0  Capacitance=c0  Setx0=off  InitialVoltage=0  Measurements=None
  Conn1 : PMIOPort  Side=Left
  connections:
  Series RLC Branch31/LConn1 -- Series RLC Branch2/LConn1 -- Conn1/RConn1
  Series RLC Branch31/RConn1 -- Series RLC Branch2/RConn1 -- Ground/LConn1

== system Ladder_Model/Subsystem5/LC1 ==
  Ground : spsGroundLib/Ground  LConnTagsString=a
  Series RLC Branch2 : spsSeriesRLCBranchLib/Series RLC Branch  LConnTagsString=__new0  RConnTagsString=__new0  BranchType=L  Resistance=1  Inductance=1e-6  SetiL0=off  InitialCurrent=0  Capacitance=1e-6  Setx0=off  InitialVoltage=0  Measurements=None
  Series RLC Branch31 : spsSeriesRLCBranchLib/Series RLC Branch  LConnTagsString=__new0  RConnTagsString=__new0  BranchType=C  Resistance=1  Inductance=1e-6  SetiL0=off  InitialCurrent=0  Capacitance=c0  Setx0=off  InitialVoltage=0  Measurements=None
  Conn1 : PMIOPort  Side=Left
  connections:
  Series RLC Branch31/LConn1 -- Series RLC Branch2/LConn1 -- Conn1/RConn1
  Series RLC Branch31/RConn1 -- Series RLC Branch2/RConn1 -- Ground/LConn1

== system Ladder_Model/Subsystem5/LC2 ==
  Ground : spsGroundLib/Ground  LConnTagsString=a
  Series RLC Branch2 : spsSeriesRLCBranchLib/Series RLC Branch  LConnTagsString=__new0  RConnTagsString=__new0  BranchType=L  Resistance=1  Inductance=1e-6  SetiL0=off  InitialCurrent=0  Capacitance=1e-6  Setx0=off  InitialVoltage=0  Measurements=None
  Series RLC Branch31 : spsSeriesRLCBranchLib/Series RLC Branch  LConnTagsString=__new0  RConnTagsString=__new0  BranchType=C  Resistance=1  Inductance=1e-6  SetiL0=off  InitialCurrent=0  Capacitance=c0  Setx0=off  InitialVoltage=0  Measurements=None
  Conn1 : PMIOPort  Side=Left
  connections:
  Series RLC Branch31/LConn1 -- Series RLC Branch2/LConn1 -- Conn1/RConn1
  Series RLC Branch31/RConn1 -- Series RLC Branch2/RConn1 -- Ground/LConn1

== system Ladder_Model/Subsystem5/LC3 ==
  Ground : spsGroundLib/Ground  LConnTagsString=a
  Series RLC Branch2 : spsSeriesRLCBranchLib/Series RLC Branch  LConnTagsString=__new0  RConnTagsString=__new0  BranchType=L  Resistance=1  Inductance=1e-6  SetiL0=off  InitialCurrent=0  Capacitance=1e-6  Setx0=off  InitialVoltage=0  Measurements=None
  Series RLC Branch31 : spsSeriesRLCBranchLib/Series RLC Branch  LConnTagsString=__new0  RConnTagsString=__new0  BranchType=C  Resistance=1  Inductance=1e-6  SetiL0=off  InitialCurrent=0  Capacitance=c0  Setx0=off  InitialVoltage=0  Measurements=None
  Conn1 : PMIOPort  Side=Left
  connections:
  Series RLC Branch31/LConn1 -- Series RLC Branch2/LConn1 -- Conn1/RConn1
  Series RLC Branch31/RConn1 -- Series RLC Branch2/RConn1 -- Ground/LConn1

== system Ladder_Model/Subsystem6/LC0 ==
  Ground : spsGroundLib/Ground  LConnTagsString=a
  Series RLC Branch2 : spsSeriesRLCBranchLib/Series RLC Branch  LConnTagsString=__new0  RConnTagsString=__new0  BranchType=L  Resistance=1  Inductance=1e-6  SetiL0=off  InitialCurrent=0  Capacitance=1e-6  Setx0=off  InitialVoltage=0  Measurements=None
  Series RLC Branch31 : spsSeriesRLCBranchLib/Series RLC Branch  LConnTagsString=__new0  RConnTagsString=__new0  BranchType=C  Resistance=1  Inductance=1e-6  SetiL0=off  InitialCurrent=0  Capacitance=c0  Setx0=off  InitialVoltage=0  Measurements=None
  Conn1 : PMIOPort  Side=Left
  connections:
  Series RLC Branch31/LConn1 -- Series RLC Branch2/LConn1 -- Conn1/RConn1
  Series RLC Branch31/RConn1 -- Series RLC Branch2/RConn1 -- Ground/LConn1

== system Ladder_Model/Subsystem6/LC1 ==
  Ground : spsGroundLib/Ground  LConnTagsString=a
  Series RLC Branch2 : spsSeriesRLCBranchLib/Series RLC Branch  LConnTagsString=__new0  RConnTagsString=__new0  BranchType=L  Resistance=1  Inductance=1e-6  SetiL0=off  InitialCurrent=0  Capacitance=1e-6  Setx0=off  InitialVoltage=0  Measurements=None
  Series RLC Branch31 : spsSeriesRLCBranchLib/Series RLC Branch  LConnTagsString=__new0  RConnTagsString=__new0  BranchType=C  Resistance=1  Inductance=1e-6  SetiL0=off  InitialCurrent=0  Capacitance=c0  Setx0=off  InitialVoltage=0  Measurements=None
  Conn1 : PMIOPort  Side=Left
  connections:
  Series RLC Branch31/LConn1 -- Series RLC Branch2/LConn1 -- Conn1/RConn1
  Series RLC Branch31/RConn1 -- Series RLC Branch2/RConn1 -- Ground/LConn1

== system Ladder_Model/Subsystem6/LC2 ==
  Ground : spsGroundLib/Ground  LConnTagsString=a
  Series RLC Branch2 : spsSeriesRLCBranchLib/Series RLC Branch  LConnTagsString=__new0  RConnTagsString=__new0  BranchType=L  Resistance=1  Inductance=1e-6  SetiL0=off  InitialCurrent=0  Capacitance=1e-6  Setx0=off  InitialVoltage=0  Measurements=None
  Series RLC Branch31 : spsSeriesRLCBranchLib/Series RLC Branch  LConnTagsString=__new0  RConnTagsString=__new0  BranchType=C  Resistance=1  Inductance=1e-6  SetiL0=off  InitialCurrent=0  Capacitance=c0  Setx0=off  InitialVoltage=0  Measurements=None
  Conn1 : PMIOPort  Side=Left
  connections:
  Series RLC Branch31/LConn1 -- Series RLC Branch2/LConn1 -- Conn1/RConn1
  Series RLC Branch31/RConn1 -- Series RLC Branch2/RConn1 -- Ground/LConn1

== system Ladder_Model/Subsystem6/LC3 ==
  Ground : spsGroundLib/Ground  LConnTagsString=a
  Series RLC Branch2 : spsSeriesRLCBranchLib/Series RLC Branch  LConnTagsString=__new0  RConnTagsString=__new0  BranchType=L  Resistance=1  Inductance=1e-6  SetiL0=off  InitialCurrent=0  Capacitance=1e-6  Setx0=off  InitialVoltage=0  Measurements=None
  Series RLC Branch31 : spsSeriesRLCBranchLib/Series RLC Branch  LConnTagsString=__new0  RConnTagsString=__new0  BranchType=C  Resistance=1  Inductance=1e-6  SetiL0=off  InitialCurrent=0  Capacitance=c0  Setx0=off  InitialVoltage=0  Measurements=None
  Conn1 : PMIOPort  Side=Left
  connections:
  Series RLC Branch31/LConn1 -- Series RLC Branch2/LConn1 -- Conn1/RConn1
  Series RLC Branch31/RConn1 -- Series RLC Branch2/RConn1 -- Ground/LConn1

== system Ladder_Model/Subsystem7/LC0 ==
  Ground : spsGroundLib/Ground  LConnTagsString=a
  Series RLC Branch2 : spsSeriesRLCBranchLib/Series RLC Branch  LConnTagsString=__new0  RConnTagsString=__new0  BranchType=L  Resistance=1  Inductance=1e-6  SetiL0=off  InitialCurrent=0  Capacitance=1e-6  Setx0=off  InitialVoltage=0  Measurements=None
  Series RLC Branch31 : spsSeriesRLCBranchLib/Series RLC Branch  LConnTagsString=__new0  RConnTagsString=__new0  BranchType=C  Resistance=1  Inductance=1e-6  SetiL0=off  InitialCurrent=0  Capacitance=c0  Setx0=off  InitialVoltage=0  Measurements=None
  Conn1 : PMIOPort  Side=Left
  connections:
  Series RLC Branch31/LConn1 -- Series RLC Branch2/LConn1 -- Conn1/RConn1
  Series RLC Branch31/RConn1 -- Series RLC Branch2/RConn1 -- Ground/LConn1

== system Ladder_Model/Subsystem7/LC1 ==
  Ground : spsGroundLib/Ground  LConnTagsString=a
  Series RLC Branch2 : spsSeriesRLCBranchLib/Series RLC Branch  LConnTagsString=__new0  RConnTagsString=__new0  BranchType=L  Resistance=1  Inductance=1e-6  SetiL0=off  InitialCurrent=0  Capacitance=1e-6  Setx0=off  InitialVoltage=0  Measurements=None
  Series RLC Branch31 : spsSeriesRLCBranchLib/Series RLC Branch  LConnTagsString=__new0  RConnTagsString=__new0  BranchType=C  Resistance=1  Inductance=1e-6  SetiL0=off  InitialCurrent=0  Capacitance=c0  Setx0=off  InitialVoltage=0  Measurements=None
  Conn1 : PMIOPort  Side=Left
  connections:
  Series RLC Branch31/LConn1 -- Series RLC Branch2/LConn1 -- Conn1/RConn1
  Series RLC Branch31/RConn1 -- Series RLC Branch2/RConn1 -- Ground/LConn1

== system Ladder_Model/Subsystem7/LC2 ==
  Ground : spsGroundLib/Ground  LConnTagsString=a
  Series RLC Branch2 : spsSeriesRLCBranchLib/Series RLC Branch  LConnTagsString=__new0  RConnTagsString=__new0  BranchType=L  Resistance=1  Inductance=1e-6  SetiL0=off  InitialCurrent=0  Capacitance=1e-6  Setx0=off  InitialVoltage=0  Measurements=None
  Series RLC Branch31 : spsSeriesRLCBranchLib/Series RLC Branch  LConnTagsString=__new0  RConnTagsString=__new0  BranchType=C  Resistance=1  Inductance=1e-6  SetiL0=off  InitialCurrent=0  Capacitance=c0  Setx0=off  InitialVoltage=0  Measurements=None
  Conn1 : PMIOPort  Side=Left
  connections:
  Series RLC Branch31/LConn1 -- Series RLC Branch2/LConn1 -- Conn1/RConn1
  Series RLC Branch31/RConn1 -- Series RLC Branch2/RConn1 -- Ground/LConn1

== system Ladder_Model/Subsystem7/LC3 ==
  Ground : spsGroundLib/Ground  LConnTagsString=a
  Series RLC Branch2 : spsSeriesRLCBranchLib/Series RLC Branch  LConnTagsString=__new0  RConnTagsString=__new0  BranchType=L  Resistance=1  Inductance=1e-6  SetiL0=off  InitialCurrent=0  Capacitance=1e-6  Setx0=off  InitialVoltage=0  Measurements=None
  Series RLC Branch31 : spsSeriesRLCBranchLib/Series RLC Branch  LConnTagsString=__new0  RConnTagsString=__new0  BranchType=C  Resistance=1  Inductance=1e-6  SetiL0=off  InitialCurrent=0  Capacitance=c0  Setx0=off  InitialVoltage=0  Measurements=None
  Conn1 : PMIOPort  Side=Left
  connections:
  Series RLC Branch31/LConn1 -- Series RLC Branch2/LConn1 -- Conn1/RConn1
  Series RLC Branch31/RConn1 -- Series RLC Branch2/RConn1 -- Ground/LConn1

== system Ladder_Model/Subsystem8/LC0 ==
  Ground : spsGroundLib/Ground  LConnTagsString=a
  Series RLC Branch2 : spsSeriesRLCBranchLib/Series RLC Branch  LConnTagsString=__new0  RConnTagsString=__new0  BranchType=L  Resistance=1  Inductance=1e-6  SetiL0=off  InitialCurrent=0  Capacitance=1e-6  Setx0=off  InitialVoltage=0  Measurements=None
  Series RLC Branch31 : spsSeriesRLCBranchLib/Series RLC Branch  LConnTagsString=__new0  RConnTagsString=__new0  BranchType=C  Resistance=1  Inductance=1e-6  SetiL0=off  InitialCurrent=0  Capacitance=c0  Setx0=off  InitialVoltage=0  Measurements=None
  Conn1 : PMIOPort  Side=Left
  connections:
  Series RLC Branch31/LConn1 -- Series RLC Branch2/LConn1 -- Conn1/RConn1
  Series RLC Branch31/RConn1 -- Series RLC Branch2/RConn1 -- Ground/LConn1

== system Ladder_Model/Subsystem8/LC1 ==
  Ground : spsGroundLib/Ground  LConnTagsString=a
  Series RLC Branch2 : spsSeriesRLCBranchLib/Series RLC Branch  LConnTagsString=__new0  RConnTagsString=__new0  BranchType=L  Resistance=1  Inductance=1e-6  SetiL0=off  InitialCurrent=0  Capacitance=1e-6  Setx0=off  InitialVoltage=0  Measurements=None
  Series RLC Branch31 : spsSeriesRLCBranchLib/Series RLC Branch  LConnTagsString=__new0  RConnTagsString=__new0  BranchType=C  Resistance=1  Inductance=1e-6  SetiL0=off  InitialCurrent=0  Capacitance=c0  Setx0=off  InitialVoltage=0  Measurements=None
  Conn1 : PMIOPort  Side=Left
  connections:
  Series RLC Branch31/LConn1 -- Series RLC Branch2/LConn1 -- Conn1/RConn1
  Series RLC Branch31/RConn1 -- Series RLC Branch2/RConn1 -- Ground/LConn1

== system Ladder_Model/Subsystem8/LC2 ==
  Ground : spsGroundLib/Ground  LConnTagsString=a
  Series RLC Branch2 : spsSeriesRLCBranchLib/Series RLC Branch  LConnTagsString=__new0  RConnTagsString=__new0  BranchType=L  Resistance=1  Inductance=1e-6  SetiL0=off  InitialCurrent=0  Capacitance=1e-6  Setx0=off  InitialVoltage=0  Measurements=None
  Series RLC Branch31 : spsSeriesRLCBranchLib/Series RLC Branch  LConnTagsString=__new0  RConnTagsString=__new0  BranchType=C  Resistance=1  Inductance=1e-6  SetiL0=off  InitialCurrent=0  Capacitance=c0  Setx0=off  InitialVoltage=0  Measurements=None
  Conn1 : PMIOPort  Side=Left
  connections:
  Series RLC Branch31/LConn1 -- Series RLC Branch2/LConn1 -- Conn1/RConn1
  Series RLC Branch31/RConn1 -- Series RLC Branch2/RConn1 -- Ground/LConn1

== system Ladder_Model/Subsystem8/LC3 ==
  Ground : spsGroundLib/Ground  LConnTagsString=a
  Series RLC Branch2 : spsSeriesRLCBranchLib/Series RLC Branch  LConnTagsString=__new0  RConnTagsString=__new0  BranchType=L  Resistance=1  Inductance=1e-6  SetiL0=off  InitialCurrent=0  Capacitance=1e-6  Setx0=off  InitialVoltage=0  Measurements=None
  Series RLC Branch31 : spsSeriesRLCBranchLib/Series RLC Branch  LConnTagsString=__new0  RConnTagsString=__new0  BranchType=C  Resistance=1  Inductance=1e-6  SetiL0=off  InitialCurrent=0  Capacitance=c0  Setx0=off  InitialVoltage=0  Measurements=None
  Conn1 : PMIOPort  Side=Left
  connections:
  Series RLC Branch31/LConn1 -- Series RLC Branch2/LConn1 -- Conn1/RConn1
  Series RLC Branch31/RConn1 -- Series RLC Branch2/RConn1 -- Ground/LConn1

== system Ladder_Model/Subsystem9/LC0 ==
  Ground : spsGroundLib/Ground  LConnTagsString=a
  Series RLC Branch2 : spsSeriesRLCBranchLib/Series RLC Branch  LConnTagsString=__new0  RConnTagsString=__new0  BranchType=L  Resistance=1  Inductance=1e-6  SetiL0=off  InitialCurrent=0  Capacitance=1e-6  Setx0=off  InitialVoltage=0  Measurements=None
  Series RLC Branch31 : spsSeriesRLCBranchLib/Series RLC Branch  LConnTagsString=__new0  RConnTagsString=__new0  BranchType=C  Resistance=1  Inductance=1e-6  SetiL0=off  InitialCurrent=0  Capacitance=c0  Setx0=off  InitialVoltage=0  Measurements=None
  Conn1 : PMIOPort  Side=Left
  connections:
  Series RLC Branch31/LConn1 -- Series RLC Branch2/LConn1 -- Conn1/RConn1
  Series RLC Branch31/RConn1 -- Series RLC Branch2/RConn1 -- Ground/LConn1

== system Ladder_Model/Subsystem9/LC1 ==
  Ground : spsGroundLib/Ground  LConnTagsString=a
  Series RLC Branch2 : spsSeriesRLCBranchLib/Series RLC Branch  LConnTagsString=__new0  RConnTagsString=__new0  BranchType=L  Resistance=1  Inductance=1e-6  SetiL0=off  InitialCurrent=0  Capacitance=1e-6  Setx0=off  InitialVoltage=0  Measurements=None
  Series RLC Branch31 : spsSeriesRLCBranchLib/Series RLC Branch  LConnTagsString=__new0  RConnTagsString=__new0  BranchType=C  Resistance=1  Inductance=1e-6  SetiL0=off  InitialCurrent=0  Capacitance=c0  Setx0=off  InitialVoltage=0  Measurements=None
  Conn1 : PMIOPort  Side=Left
  connections:
  Series RLC Branch31/LConn1 -- Series RLC Branch2/LConn1 -- Conn1/RConn1
  Series RLC Branch31/RConn1 -- Series RLC Branch2/RConn1 -- Ground/LConn1

== system Ladder_Model/Subsystem9/LC2 ==
  Ground : spsGroundLib/Ground  LConnTagsString=a
  Series RLC Branch2 : spsSeriesRLCBranchLib/Series RLC Branch  LConnTagsString=__new0  RConnTagsString=__new0  BranchType=L  Resistance=1  Inductance=1e-6  SetiL0=off  InitialCurrent=0  Capacitance=1e-6  Setx0=off  InitialVoltage=0  Measurements=None
  Series RLC Branch31 : spsSeriesRLCBranchLib/Series RLC Branch  LConnTagsString=__new0  RConnTagsString=__new0  BranchType=C  Resistance=1  Inductance=1e-6  SetiL0=off  InitialCurrent=0  Capacitance=c0  Setx0=off  InitialVoltage=0  Measurements=None
  Conn1 : PMIOPort  Side=Left
  connections:
  Series RLC Branch31/LConn1 -- Series RLC Branch2/LConn1 -- Conn1/RConn1
  Series RLC Branch31/RConn1 -- Series RLC Branch2/RConn1 -- Ground/LConn1

== system Ladder_Model/Subsystem9/LC3 ==
  Ground : spsGroundLib/Ground  LConnTagsString=a
  Series RLC Branch2 : spsSeriesRLCBranchLib/Series RLC Branch  LConnTagsString=__new0  RConnTagsString=__new0  BranchType=L  Resistance=1  Inductance=1e-6  SetiL0=off  InitialCurrent=0  Capacitance=1e-6  Setx0=off  InitialVoltage=0  Measurements=None
  Series RLC Branch31 : spsSeriesRLCBranchLib/Series RLC Branch  LConnTagsString=__new0  RConnTagsString=__new0  BranchType=C  Resistance=1  Inductance=1e-6  SetiL0=off  InitialCurrent=0  Capacitance=c0  Setx0=off  InitialVoltage=0  Measurements=None
  Conn1 : PMIOPort  Side=Left
  connections:
  Series RLC Branch31/LConn1 -- Series RLC Branch2/LConn1 -- Conn1/RConn1
  Series RLC Branch31/RConn1 -- Series RLC Branch2/RConn1 -- Ground/LConn1
